simulink model "SuspensionEffectsOnCornering"  (R2024a)
settings: Solver=VariableStepAuto  StartTime=0.0  StopTime=Sim_Time  MaxStep=0.02  RelTol=1e-3
values from neighbouring files (symbols this model uses):
  b = 3000    [SuspensionEffectsOnCorneringRun.m]
  BackLeftLateral = 1225    [SuspensionEffectsOnCorneringRun.m]
  BackRightLateral = 1200    [SuspensionEffectsOnCorneringRun.m]
  CurvatureRadius = 600    [SuspensionEffectsOnCorneringRun.m]
  FrontLeftLateral = 1650    [SuspensionEffectsOnCorneringRun.m]
  FrontRightLateral = 1600    [SuspensionEffectsOnCorneringRun.m]
  g = 9.81    [SuspensionEffectsOnCorneringRun.m]
  h1 = 0.45    [SuspensionEffectsOnCorneringRun.m]
  hr = 0.1    [SuspensionEffectsOnCorneringRun.m]
  k = 100000    [SuspensionEffectsOnCorneringRun.m]
  M = 275    [SuspensionEffectsOnCorneringRun.m]
  SeparationBetweenSprings = 1.475    [SuspensionEffectsOnCorneringRun.m]
  SpringLength = 0.4    [SuspensionEffectsOnCorneringRun.m]
  TrackWidth = 1.5    [SuspensionEffectsOnCorneringRun.m]
  VehicleMass = 1100    [SuspensionEffectsOnCorneringRun.m]
libraries: simulink_extras x1
settings Model: Creator=msi-nb  LastModifiedBy=msi-nb

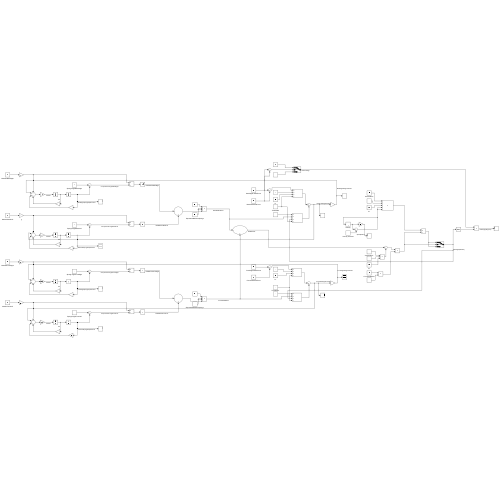
[thumbnail: Simulink's stored preview of the top-level diagram]
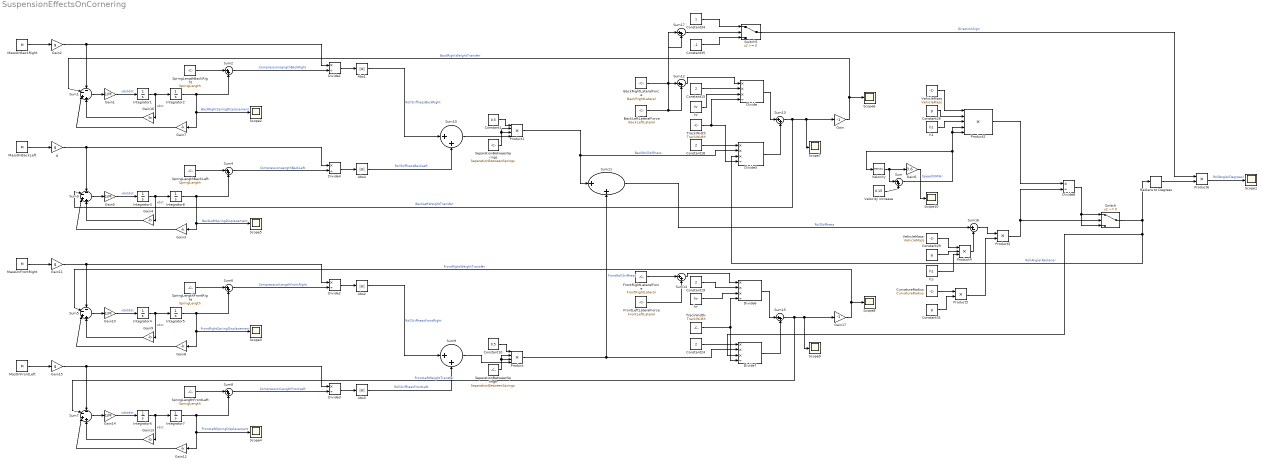
== system SuspensionEffectsOnCornering ==
  Abs{1..4} (4 alike) : Abs  SaturateOnIntegerOverflow=off
  BackLeftLateralForce : Constant  Value=BackLeftLateral
  BackRightLateralForce : Constant  Value=BackRightLateral
  Constant1 : Constant  Value=0.5
  Constant10 : Constant  Value=0.5
  Constant{15,18..19,24} (4 alike) : Constant  Value=2
  Constant26 : Constant  Value=g
  Constant29 : Constant  Value=g
  Constant31 : Constant  Value=g
  Constant34 : Constant
  Constant35 : Constant  Value=-1
  CurvatureRadius : Constant  Value=CurvatureRadius
  Divide{,5..7} (4 alike) : Product  Inputs=***/
  Divide{1..4,8} (5 alike) : Product  Inputs=*/
  FrontLeftLateralForce : Constant  Value=FrontLeftLateral
  FrontRightLateralForce : Constant  Value=FrontRightLateral
  Gain : Gain  Gain=-1
  Gain{1,5,10,14} (4 alike) : Gain  Gain=1/M
  Gain11 : Gain  Gain=g
  Gain{3,7..8,12} (4 alike) : Gain  Gain=-k
  Gain{4,9,13,16} (4 alike) : Gain  Gain=-b
  Gain15 : Gain  Gain=g
  Gain17 : Gain  Gain=-1
  Gain2 : Gain  Gain=g
  Gain6 : Gain  Gain=3.6
  Integrator{1..8} (8 alike) : Integrator
  MasOnFrontLeft : Constant  Value=M
  MassOnBackLeft : Constant  Value=M
  MassOnBackRight : Constant  Value=M
  MassOnFrontRight : Constant  Value=M
  Product : Product  Inputs=4
  Product1 : Product  Inputs=4
  Product2 : Product  Inputs=5
  Product3 : Product
  Product4 : Product  Inputs=3
  Product5 : Product
  Product6 : Product
  Radians to Degrees : simulink_extras/Transformations/Radians to Degrees
  Scope{1..10} (10 alike) : Scope
  SeparationBetweenSprings : Constant  Value=SeparationBetweenSprings
  SeparationBetweenSprings- : Constant  Value=SeparationBetweenSprings
  SpringLengthBackLeft : Constant  Value=SpringLength
  SpringLengthBackRight : Constant  Value=SpringLength
  SpringLengthFrontLeft : Constant  Value=SpringLength
  SpringLengthFrontRight : Constant  Value=SpringLength
  Sum{,2,4,6,8..15,17} (13 alike) : Sum  Inputs=|++
  Sum{1,3,5,7} (4 alike) : Sum  Inputs=--++
  Sum16 : Sum  Inputs=|+-
  Switch : Switch  Criteria=u2 ~= 0  SaturateOnIntegerOverflow=off  InputSameDT=off
  Switch5 : Switch  SaturateOnIntegerOverflow=off  InputSameDT=off
  TrackWidth : Constant  Value=TrackWidth
  TrackWidth- : Constant  Value=TrackWidth
  VehicleMass : Constant  Value=VehicleMass
  VehicleMass- : Constant  Value=VehicleMass
  Velocity : Memory  InitialCondition=25
  Velocity increase : Constant  Value=0.15
  g : Gain  Gain=g
  h1 : Constant  Value=h1
  h1- : Constant  Value=h1
  hr : Constant  Value=hr
  hr- : Constant  Value=hr
  wires:
  Velocity/1 -> Gain6/1, Sum/1
  Velocity increase/1 -> Sum/2
  Sum/1 -> Product2/5, Product2/4, Velocity/1
  Integrator6/1 -> Gain13/1, Integrator7/1  "xdot"
  Gain14/1 -> Integrator6/1  "xdotdot"
  Abs3/1 -> Sum9/2  "RollStiffnessFrontLeft"
  Gain15/1 -> Divide3/1, Sum7/1
  Integrator7/1 -> Sum8/2, Scope4/1, Gain12/1  "FrontLeftSpringDisplacement"
  MasOnFrontLeft/1 -> Gain15/1
  Abs2/1 -> Sum9/1  "RollStiffnessFrontRight"
  Gain12/1 -> Sum7/3
  Divide2/1 -> Abs2/1
  MassOnFrontRight/1 -> Gain11/1
  SpringLengthFrontLeft/1 -> Sum8/1
  Gain9/1 -> Sum5/4
  Sum8/1 -> Divide3/2  "CompressionLengthFrontLeft"
  Gain8/1 -> Sum5/3
  Integrator5/1 -> Sum6/2, Scope3/1, Gain8/1  "FrontRightSpringDisplacement"
  Sum7/1 -> Gain14/1
  Gain11/1 -> Sum5/1, Divide2/1
  Integrator4/1 -> Gain9/1, Integrator5/1  "xdot"
  Gain10/1 -> Integrator4/1  "xdotdot"
  Sum5/1 -> Gain10/1
  SpringLengthFrontRight/1 -> Sum6/1
  Sum6/1 -> Divide2/2  "CompressionLengthFrontRight"
  Divide3/1 -> Abs3/1
  Gain13/1 -> Sum7/4
  SeparationBetweenSprings-/1 -> Product/2, Product/3
  Sum9/1 -> Product/4
  Constant10/1 -> Product/1
  Product/1 -> Sum11/2, Divide7/2  "FrontRollStiffness"
  Abs1/1 -> Sum10/1  "RollStiffnessBackRight"
  Integrator8/1 -> Sum4/2, Scope5/1, Gain3/1  "BackLeftSpringDisplacement"
  Gain3/1 -> Sum3/3
  Sum10/1 -> Product1/4
  g/1 -> Sum3/1, Divide4/1
  Gain5/1 -> Integrator3/1  "xdotdot"
  Gain4/1 -> Sum3/4
  Divide4/1 -> Abs4/1
  Sum2/1 -> Divide1/2  "CompressionLengthBackRight"
  Sum1/1 -> Gain1/1
  SpringLengthBackRight/1 -> Sum2/1
  Gain1/1 -> Integrator1/1  "xdotdot"
  Integrator1/1 -> Gain16/1, Integrator2/1  "xdot"
  Integrator2/1 -> Sum2/2, Scope2/1, Gain7/1  "BackRightSpringDisplacement"
  Product1/1 -> Sum11/1, Divide5/2  "BackRollStiffness"
  Sum3/1 -> Gain5/1
  Gain2/1 -> Sum1/1, Divide1/1
  Integrator3/1 -> Gain4/1, Integrator8/1  "xdot"
  MassOnBackRight/1 -> Gain2/1
  Constant1/1 -> Product1/1
  Gain7/1 -> Sum1/3
  Divide1/1 -> Abs1/1
  Gain16/1 -> Sum1/4
  Sum4/1 -> Divide4/2  "CompressionLengthBackLeft"
  SpringLengthBackLeft/1 -> Sum4/1
  MassOnBackLeft/1 -> g/1
  SeparationBetweenSprings/1 -> Product1/2, Product1/3
  Abs4/1 -> Sum10/2  "RollStiffnessBackLeft"
  Sum11/1 -> Sum16/1  "RollStiffness"
  BackRightLateralForce/1 -> Sum12/1, Sum17/1
  BackLeftLateralForce/1 -> Sum17/2, Sum12/2
  Constant15/1 -> Divide/2
  Sum12/1 -> Divide/1
  hr/1 -> Divide/3
  TrackWidth/1 -> Divide5/4, Divide/4
  Constant18/1 -> Divide5/1
  Divide/1 -> Sum13/1
  Divide5/1 -> Sum13/2
  Sum13/1 -> Sum3/2, Scope7/1, Gain/1  "BackLeftWeightTransfer"
  Gain/1 -> Scope6/1, Sum1/2  "BackRightWeightTransfer"
  FrontRightLateralForce/1 -> Sum14/1
  FrontLeftLateralForce/1 -> Sum14/2
  Constant19/1 -> Divide6/2
  Sum14/1 -> Divide6/1
  hr-/1 -> Divide6/3
  TrackWidth-/1 -> Divide7/4, Divide6/4
  Divide6/1 -> Sum15/1
  Divide7/1 -> Sum15/2
  Constant24/1 -> Divide7/1
  Switch/1 -> Radians to Degrees/1, Divide7/3, Divide5/3  "RollAngle(Radians)"
  Sum15/1 -> Scope9/1, Gain17/1, Sum7/2  "FrontLeftWeightTransfer"
  Gain17/1 -> Scope8/1, Sum5/2  "FrontRightWeightTransfer"
  VehicleMass/1 -> Product2/1
  Constant26/1 -> Product2/2
  h1/1 -> Product2/3
  Product2/1 -> Divide8/1
  VehicleMass-/1 -> Product4/1
  Constant29/1 -> Product4/2
  h1-/1 -> Product4/3
  Product4/1 -> Sum16/2
  Sum16/1 -> Product3/1
  CurvatureRadius/1 -> Product5/1
  Constant31/1 -> Product5/2
  Product5/1 -> Product3/2
  Product3/1 -> Divide8/2, Switch/2
  Divide8/1 -> Switch/3, Switch/1
  Sum17/1 -> Switch5/2
  Constant34/1 -> Switch5/1
  Constant35/1 -> Switch5/3
  Radians to Degrees/1 -> Product6/2
  Switch5/1 -> Product6/1  "DirectionSign"
  Product6/1 -> Scope1/1  "RollAngle(Degrees)"
  Gain6/1 -> Scope10/1  "Speed(KM/H)"
